simulink model "SysGenBCM_MR0"  (R2015b)
settings: Solver=ode45  StartTime=0.0  StopTime=2e-3  MaxStep=100e-6  RelTol=1e-3
undefined symbols (not defined in the file): AXI4, Lite
libraries: xbsIndex_r4 x89
settings Model: DataTypeOverride=Double  MinMaxOverflowLogging=MinMaxAndOverflow  FPTRunName=DoubleOverride  Creator=ssmith  LastModifiedBy=leosap
settings DataIOCC: SaveFormat=Array
settings DebuggingCC: UnderspecifiedInitializationDetection=Classic  MergeDetectMultiDrivingBlocksExec=none  SolverPrmCheckMsg=warning
settings HardwareCC: ProdBitPerPointer=32  ProdLargestAtomicFloat=None  ProdIntDivRoundTo=Undefined  ProdEndianess=Unspecified  ProdWordSize=32  ProdHWDeviceType=32-bit Generic
settings GRTTargetCC: GeneratePreprocessorConditionals=Disable all
settings ConfigComp: CovModelRefEnable=Off  CovSFcnEnable=off

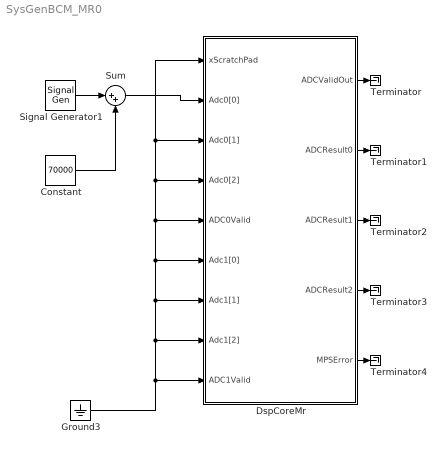
== system SysGenBCM_MR0 ==
  Constant : Constant  Value=70000
  DspCoreMr : Subsystem
  Ground3 : Ground
  Signal Generator1 : SignalGenerator  Amplitude=65000  Frequency=1E+6  Units=rad/sec
  Sum : Sum  Inputs=|++
  Terminator{,1..4} (5 alike) : Terminator
  wires:
  Ground3/1 -> DspCoreMr/9(ADC1Valid), DspCoreMr/8(Adc1[2]), DspCoreMr/7(Adc1[1]), DspCoreMr/6(Adc1[0]), DspCoreMr/3(Adc0[1]), DspCoreMr/1(xScratchPad), DspCoreMr/4(Adc0[2]), DspCoreMr/5(ADC0Valid)
  Constant/1 -> Sum/2
  Signal Generator1/1 -> Sum/1
  Sum/1 -> DspCoreMr/2(Adc0[0])
  DspCoreMr/1(ADCValidOut) -> Terminator/1
  DspCoreMr/2(ADCResult0) -> Terminator1/1
  DspCoreMr/3(ADCResult1) -> Terminator2/1
  DspCoreMr/4(ADCResult2) -> Terminator3/1
  DspCoreMr/5(MPSError) -> Terminator4/1

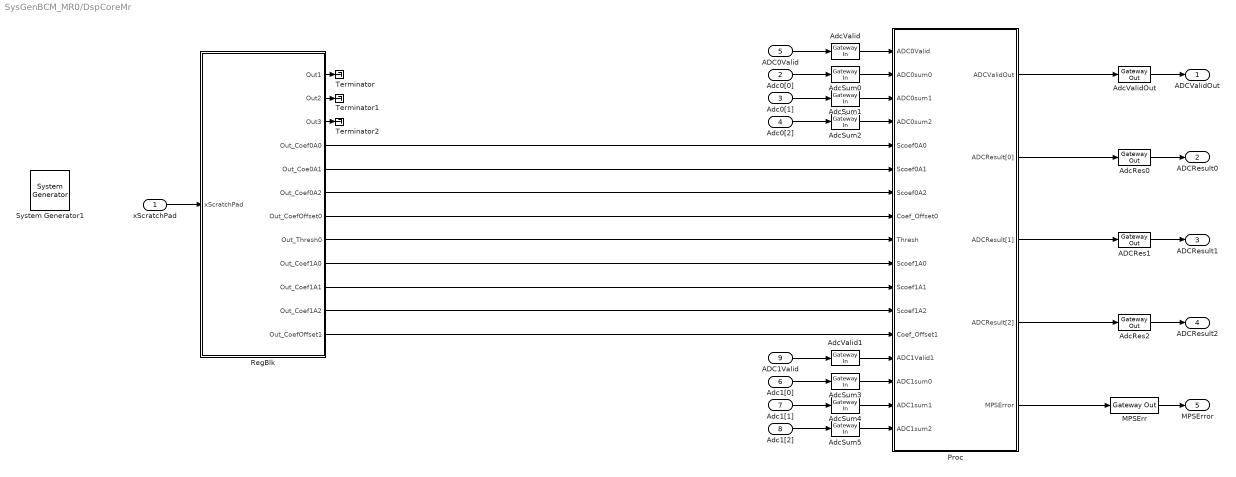
== system SysGenBCM_MR0/DspCoreMr ==
  xScratchPad : Inport
  Adc0[0] : Inport  Port=2
  Adc0[1] : Inport  Port=3
  Adc0[2] : Inport  Port=4
  ADC0Valid : Inport  Port=5
  Adc1[0] : Inport  Port=6
  Adc1[1] : Inport  Port=7
  Adc1[2] : Inport  Port=8
  ADC1Valid : Inport  Port=9
  " System Generator1" : xbsIndex_r4/ System Generator  Tag=genX  xilinxfamily=kintexu  part=xcku040  speed=-2-e  package=ffva1156  synthesis_tool=Vivado  clock_wrapper=Clock Enables  directory=./netlist  proj_type=Vivado  Synth_file=Vivado Synthesis Defaults  Impl_file=Vivado Implementation Defaults  testbench=off  simulink_period=5.385e-9  sysclk_period=5.385  dcm_input_clock_period=10  incr_netlist=off  trim_vbits=Everywhere in SubSystem  dbl_ovrd=According to Block Masks  core_generation=According to Block Masks  run_coregen=off  deprecated_control=off  eval_field=0  block_type=sysgen
  ADCRes1 : xbsIndex_r4/Gateway Out  inherit_from_input=on  hdl_port=on  rows=1  columns=1  UseAsDAC=off  DACChannel='1'  interface=None  automatic_assignment=on  address_offset=hex2dec('00')  intf_name=''  intf_description=''  timing_constraint=None  locs_specified=off  LOCs={}  io_standard={}  block_type=gatewayout
  AdcRes0 : xbsIndex_r4/Gateway Out  inherit_from_input=on  hdl_port=on  rows=1  columns=1  UseAsDAC=off  DACChannel='1'  interface=None  automatic_assignment=on  address_offset=hex2dec('00')  intf_name=''  intf_description=''  timing_constraint=None  locs_specified=off  LOCs={}  io_standard={}  block_type=gatewayout
  AdcRes2 : xbsIndex_r4/Gateway Out  inherit_from_input=on  hdl_port=on  rows=1  columns=1  UseAsDAC=off  DACChannel='1'  interface=None  automatic_assignment=on  address_offset=hex2dec('00')  intf_name=''  intf_description=''  timing_constraint=None  locs_specified=off  LOCs={}  io_standard={}  block_type=gatewayout
  AdcSum{0..5} (6 alike) : xbsIndex_r4/Gateway In  gui_display_data_type=Fixed-point  arith_type=Unsigned  n_bits=32  bin_pt=0  preci_type=Single  exp_width=8  frac_width=24  rows=1  columns=1  quantization="Round  (unbiased: +/- Inf)"  overflow=Saturate  period=5.385E-9  UseAsADC=off  ADCChannel='1'  interface=None  automatic_assignment=on  address_offset=hex2dec('00')  intf_name=''  intf_description=''  default_value=0  timing_constraint=None  locs_specified=off  LOCs={}  io_standard={}  inherit_from_input=off  hdl_port=on  dbl_ovrd=off  block_type=gatewayin
  AdcValid : xbsIndex_r4/Gateway In  gui_display_data_type=Boolean  arith_type=Boolean  n_bits=1  bin_pt=0  preci_type=Single  exp_width=8  frac_width=24  rows=1  columns=1  quantization="Round  (unbiased: +/- Inf)"  overflow=Saturate  period=5.385E-9  UseAsADC=off  ADCChannel='1'  interface=None  automatic_assignment=on  address_offset=hex2dec('00')  intf_name=''  intf_description=''  default_value=0  timing_constraint=None  locs_specified=off  LOCs={}  io_standard={}  inherit_from_input=off  hdl_port=on  dbl_ovrd=off  block_type=gatewayin
  AdcValid1 : xbsIndex_r4/Gateway In  gui_display_data_type=Boolean  arith_type=Boolean  n_bits=1  bin_pt=0  preci_type=Single  exp_width=8  frac_width=24  rows=1  columns=1  quantization="Round  (unbiased: +/- Inf)"  overflow=Saturate  period=5.385E-9  UseAsADC=off  ADCChannel='1'  interface=None  automatic_assignment=on  address_offset=hex2dec('00')  intf_name=''  intf_description=''  default_value=0  timing_constraint=None  locs_specified=off  LOCs={}  io_standard={}  inherit_from_input=off  hdl_port=on  dbl_ovrd=off  block_type=gatewayin
  AdcValidOut : xbsIndex_r4/Gateway Out  inherit_from_input=on  hdl_port=on  rows=1  columns=1  UseAsDAC=off  DACChannel='1'  interface=None  automatic_assignment=on  address_offset=hex2dec('00')  intf_name=''  intf_description=''  timing_constraint=None  locs_specified=off  LOCs={}  io_standard={}  block_type=gatewayout
  MPSErr : xbsIndex_r4/Gateway Out  inherit_from_input=on  hdl_port=on  rows=1  columns=1  UseAsDAC=off  DACChannel='1'  interface=None  automatic_assignment=on  address_offset=hex2dec('00')  intf_name=''  intf_description=''  timing_constraint=None  locs_specified=off  LOCs={}  io_standard={}  block_type=gatewayout
  Proc : Subsystem
  RegBlk : Subsystem
  Terminator : Terminator
  Terminator1 : Terminator
  Terminator2 : Terminator
  ADCValidOut : Outport
  ADCResult0 : Outport  Port=2
  ADCResult1 : Outport  Port=3
  ADCResult2 : Outport  Port=4
  MPSError : Outport  Port=5
  wires:
  xScratchPad/1 -> RegBlk/1(xScratchPad)
  Proc/1(ADCValidOut) -> AdcValidOut/1
  Adc0[2]/1 -> AdcSum2/1
  Adc0[1]/1 -> AdcSum1/1
  Adc0[0]/1 -> AdcSum0/1
  Proc/3(ADCResult[1]) -> ADCRes1/1
  Proc/4(ADCResult[2]) -> AdcRes2/1
  Proc/2(ADCResult[0]) -> AdcRes0/1
  ADC0Valid/1 -> AdcValid/1
  AdcRes0/1 -> ADCResult0/1
  AdcRes2/1 -> ADCResult2/1
  ADCRes1/1 -> ADCResult1/1
  AdcValidOut/1 -> ADCValidOut/1
  AdcValid/1 -> Proc/1(ADC0Valid)
  AdcSum2/1 -> Proc/4(ADC0sum2)
  AdcSum1/1 -> Proc/3(ADC0sum1)
  AdcSum0/1 -> Proc/2(ADC0sum0)
  MPSErr/1 -> MPSError/1
  Adc1[2]/1 -> AdcSum5/1
  Adc1[1]/1 -> AdcSum4/1
  Adc1[0]/1 -> AdcSum3/1
  ADC1Valid/1 -> AdcValid1/1
  AdcValid1/1 -> Proc/14(ADC1Valid1)
  AdcSum5/1 -> Proc/17(ADC1sum2)
  AdcSum4/1 -> Proc/16(ADC1sum1)
  AdcSum3/1 -> Proc/15("ADC1sum0 ")
  RegBlk/4(Out_Coef0A0) -> Proc/5(Scoef0A0)
  RegBlk/12(Out_CoefOffset1) -> Proc/13(Coef_Offset1)
  RegBlk/5(Out_Coe0A1) -> Proc/6(Scoef0A1)
  RegBlk/6(Out_Coef0A2) -> Proc/7(Scoef0A2)
  RegBlk/7(Out_CoefOffset0) -> Proc/8(Coef_Offset0)
  RegBlk/8(Out_Thresh0) -> Proc/9(Thresh)
  RegBlk/9(Out_Coef1A0) -> Proc/10("Scoef1A0 ")
  RegBlk/10(Out_Coef1A1) -> Proc/11(Scoef1A1)
  RegBlk/11(Out_Coef1A2) -> Proc/12(Scoef1A2)
  RegBlk/1(Out1) -> Terminator/1
  RegBlk/2(Out2) -> Terminator1/1
  RegBlk/3(Out3) -> Terminator2/1
  Proc/5(MPSError) -> MPSErr/1

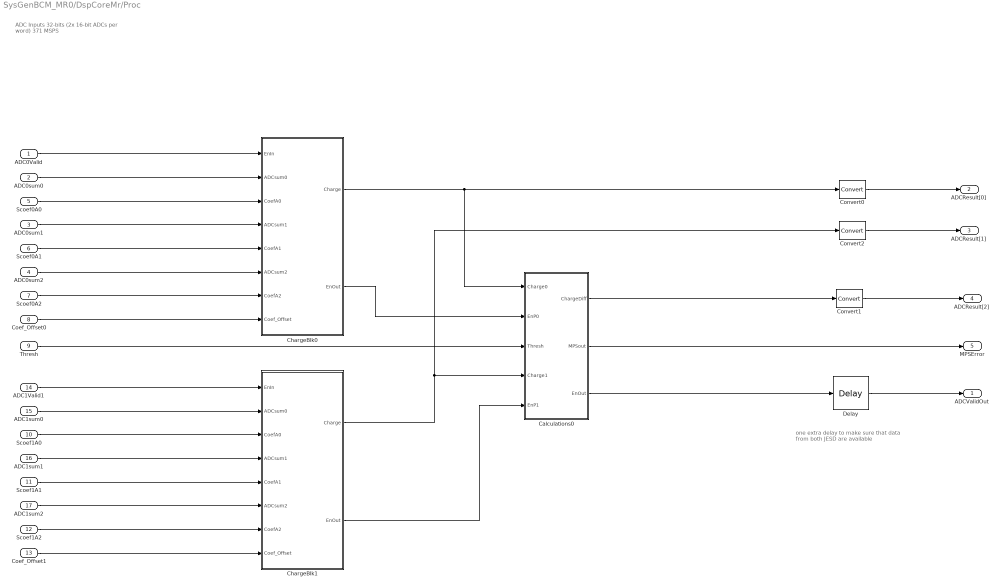
== system SysGenBCM_MR0/DspCoreMr/Proc ==
  note: ADC Inputs
      | 32-bits (2x 16-bit ADCs per word)
      | 371 MSPS
  note: one extra delay to make sure that data from both JESD are available
  ADC0Valid : Inport
  ADC0sum0 : Inport  Port=2
  ADC0sum1 : Inport  Port=3
  ADC0sum2 : Inport  Port=4
  Scoef0A0 : Inport  Port=5  SampleTime=5.385E-9
  Scoef0A1 : Inport  Port=6  SampleTime=5.385E-9
  Scoef0A2 : Inport  Port=7  SampleTime=5.385E-9
  Coef_Offset0 : Inport  Port=8  SampleTime=5.385E-9
  Thresh : Inport  Port=9  SampleTime=5.385E-9
  "Scoef1A0 " : Inport  Port=10  SampleTime=5.385E-9
  Scoef1A1 : Inport  Port=11  SampleTime=5.385E-9
  Scoef1A2 : Inport  Port=12  SampleTime=5.385E-9
  Coef_Offset1 : Inport  Port=13  SampleTime=5.385E-9
  ADC1Valid1 : Inport  Port=14
  "ADC1sum0 " : Inport  Port=15
  ADC1sum1 : Inport  Port=16
  ADC1sum2 : Inport  Port=17
  Calculations0 : Subsystem
  ChargeBlk0 : Subsystem
  ChargeBlk1 : Subsystem
  Convert0 : xbsIndex_r4/Convert  gui_display_data_type=Fixed-point  arith_type="Signed  (2's comp)"  n_bits=32  bin_pt=0  float_type=Single  exp_bits=8  fraction_bits=24  quantization="Round  (unbiased: +/- Inf)"  overflow=Saturate  en=off  latency=1  pipeline=off  dbl_ovrd=off  block_type=convert
  Convert1 : xbsIndex_r4/Convert  gui_display_data_type=Fixed-point  arith_type="Signed  (2's comp)"  n_bits=32  bin_pt=0  float_type=Single  exp_bits=8  fraction_bits=24  quantization="Round  (unbiased: +/- Inf)"  overflow=Saturate  en=off  latency=1  pipeline=off  dbl_ovrd=off  block_type=convert
  Convert2 : xbsIndex_r4/Convert  gui_display_data_type=Fixed-point  arith_type="Signed  (2's comp)"  n_bits=32  bin_pt=0  float_type=Single  exp_bits=8  fraction_bits=24  quantization="Round  (unbiased: +/- Inf)"  overflow=Saturate  en=off  latency=1  pipeline=off  dbl_ovrd=off  block_type=convert
  Delay : xbsIndex_r4/Delay  rst=off  infoeditControl=Selection of Reset will increase slice count due to use of real FFs and instead of SRLs  en=off  latency=2  reg_retiming=off  dbl_ovrd=off  block_type=delay
      settings: infoedit=Hardware notes: A delay line is a chain, each link of which is an SRL16 or SRL32 followed by a flip-flop.
  ADCValidOut : Outport
  ADCResult[0] : Outport  Port=2
  ADCResult[1] : Outport  Port=3
  ADCResult[2] : Outport  Port=4
  MPSError : Outport  Port=5
  wires:
  Convert0/1 -> ADCResult[0]/1
  Convert1/1 -> ADCResult[2]/1
  Delay/1 -> ADCValidOut/1
  Convert2/1 -> ADCResult[1]/1
  Calculations0/1(ChargeDiff) -> Convert1/1
  Calculations0/3(EnOut) -> Delay/1
  Calculations0/2(MPSout) -> MPSError/1
  Thresh/1 -> Calculations0/3(Thresh)
  ADC0Valid/1 -> ChargeBlk0/1(EnIn)
  ADC0sum0/1 -> ChargeBlk0/2(ADCsum0)
  Scoef0A0/1 -> ChargeBlk0/3(CoefA0)
  ADC0sum1/1 -> ChargeBlk0/4(ADCsum1)
  Scoef0A1/1 -> ChargeBlk0/5(CoefA1)
  ADC0sum2/1 -> ChargeBlk0/6(ADCsum2)
  Scoef0A2/1 -> ChargeBlk0/7(CoefA2)
  Coef_Offset0/1 -> ChargeBlk0/8(Coef_Offset)
  ChargeBlk0/2(EnOut) -> Calculations0/2(EnP0)
  ChargeBlk0/1(Charge) -> Calculations0/1(Charge0), Convert0/1
  ChargeBlk1/1(Charge) -> Convert2/1, Calculations0/4(Charge1)
  ChargeBlk1/2(EnOut) -> Calculations0/5(EnP1)
  ADC1Valid1/1 -> ChargeBlk1/1(EnIn)
  "ADC1sum0 "/1 -> ChargeBlk1/2(ADCsum0)
  "Scoef1A0 "/1 -> ChargeBlk1/3(CoefA0)
  ADC1sum1/1 -> ChargeBlk1/4(ADCsum1)
  Scoef1A1/1 -> ChargeBlk1/5(CoefA1)
  ADC1sum2/1 -> ChargeBlk1/6(ADCsum2)
  Scoef1A2/1 -> ChargeBlk1/7(CoefA2)
  Coef_Offset1/1 -> ChargeBlk1/8(Coef_Offset)

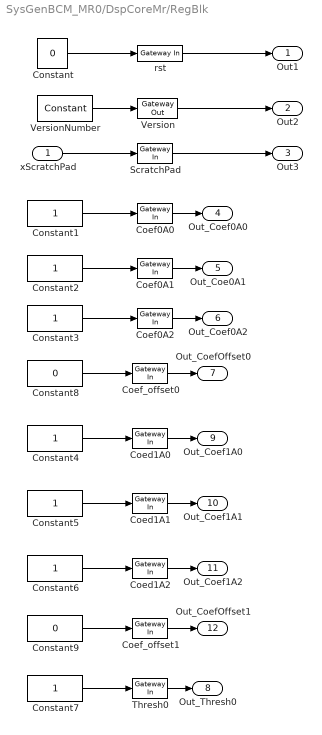
== system SysGenBCM_MR0/DspCoreMr/RegBlk ==
  xScratchPad : Inport
  Coed1A0 : xbsIndex_r4/Gateway In  gui_display_data_type=Floating-point  arith_type=Floating-point  n_bits=32  bin_pt=0  preci_type=Single  exp_width=8  frac_width=24  rows=1  columns=1  quantization="Round  (unbiased: +/- Inf)"  overflow=Saturate  period=5.385E-9  UseAsADC=off  ADCChannel='1'  interface=AXI4-Lite  automatic_assignment=off  address_offset=hex2dec('014')  intf_name='rwreg'  intf_description=''  default_value=0  timing_constraint=None  locs_specified=off  LOCs={}  io_standard={}  inherit_from_input=off  hdl_port=on  dbl_ovrd=off  block_type=gatewayin
  Coed1A1 : xbsIndex_r4/Gateway In  gui_display_data_type=Floating-point  arith_type=Floating-point  n_bits=32  bin_pt=0  preci_type=Single  exp_width=8  frac_width=24  rows=1  columns=1  quantization="Round  (unbiased: +/- Inf)"  overflow=Saturate  period=5.385E-9  UseAsADC=off  ADCChannel='1'  interface=AXI4-Lite  automatic_assignment=off  address_offset=hex2dec('018')  intf_name='rwreg'  intf_description=''  default_value=0  timing_constraint=None  locs_specified=off  LOCs={}  io_standard={}  inherit_from_input=off  hdl_port=on  dbl_ovrd=off  block_type=gatewayin
  Coed1A2 : xbsIndex_r4/Gateway In  gui_display_data_type=Floating-point  arith_type=Floating-point  n_bits=32  bin_pt=0  preci_type=Single  exp_width=8  frac_width=24  rows=1  columns=1  quantization="Round  (unbiased: +/- Inf)"  overflow=Saturate  period=5.385E-9  UseAsADC=off  ADCChannel='1'  interface=AXI4-Lite  automatic_assignment=off  address_offset=hex2dec('01C')  intf_name='rwreg'  intf_description=''  default_value=0  timing_constraint=None  locs_specified=off  LOCs={}  io_standard={}  inherit_from_input=off  hdl_port=on  dbl_ovrd=off  block_type=gatewayin
  Coef0A0 : xbsIndex_r4/Gateway In  gui_display_data_type=Floating-point  arith_type=Floating-point  n_bits=32  bin_pt=31  preci_type=Single  exp_width=8  frac_width=24  rows=1  columns=1  quantization="Round  (unbiased: +/- Inf)"  overflow=Saturate  period=5.385E-9  UseAsADC=off  ADCChannel='1'  interface=AXI4-Lite  automatic_assignment=off  address_offset=hex2dec('004')  intf_name='rwreg'  intf_description=''  default_value=hex2dec('3f800000')  timing_constraint=None  locs_specified=off  LOCs={}  io_standard={}  inherit_from_input=off  hdl_port=on  dbl_ovrd=off  block_type=gatewayin
  Coef0A1 : xbsIndex_r4/Gateway In  gui_display_data_type=Floating-point  arith_type=Floating-point  n_bits=32  bin_pt=0  preci_type=Single  exp_width=8  frac_width=24  rows=1  columns=1  quantization="Round  (unbiased: +/- Inf)"  overflow=Saturate  period=5.385E-9  UseAsADC=off  ADCChannel='1'  interface=AXI4-Lite  automatic_assignment=off  address_offset=hex2dec('008')  intf_name='rwreg'  intf_description=''  default_value=hex2dec('3f800001')  timing_constraint=None  locs_specified=off  LOCs={}  io_standard={}  inherit_from_input=off  hdl_port=on  dbl_ovrd=off  block_type=gatewayin
  Coef0A2 : xbsIndex_r4/Gateway In  gui_display_data_type=Floating-point  arith_type=Floating-point  n_bits=32  bin_pt=0  preci_type=Single  exp_width=8  frac_width=24  rows=1  columns=1  quantization="Round  (unbiased: +/- Inf)"  overflow=Saturate  period=5.385E-9  UseAsADC=off  ADCChannel='1'  interface=AXI4-Lite  automatic_assignment=off  address_offset=hex2dec('00C')  intf_name='rwreg'  intf_description=''  default_value=hex2dec('3f800002')  timing_constraint=None  locs_specified=off  LOCs={}  io_standard={}  inherit_from_input=off  hdl_port=on  dbl_ovrd=off  block_type=gatewayin
  Coef_offset0 : xbsIndex_r4/Gateway In  gui_display_data_type=Floating-point  arith_type=Floating-point  n_bits=32  bin_pt=0  preci_type=Single  exp_width=8  frac_width=24  rows=1  columns=1  quantization="Round  (unbiased: +/- Inf)"  overflow=Saturate  period=5.385E-9  UseAsADC=off  ADCChannel='1'  interface=AXI4-Lite  automatic_assignment=off  address_offset=hex2dec('010')  intf_name='rwreg'  intf_description=''  default_value=0  timing_constraint=None  locs_specified=off  LOCs={}  io_standard={}  inherit_from_input=off  hdl_port=on  dbl_ovrd=off  block_type=gatewayin
  Coef_offset1 : xbsIndex_r4/Gateway In  gui_display_data_type=Floating-point  arith_type=Floating-point  n_bits=32  bin_pt=0  preci_type=Single  exp_width=8  frac_width=24  rows=1  columns=1  quantization="Round  (unbiased: +/- Inf)"  overflow=Saturate  period=5.385E-9  UseAsADC=off  ADCChannel='1'  interface=AXI4-Lite  automatic_assignment=off  address_offset=hex2dec('020')  intf_name='rwreg'  intf_description=''  default_value=0  timing_constraint=None  locs_specified=off  LOCs={}  io_standard={}  inherit_from_input=off  hdl_port=on  dbl_ovrd=off  block_type=gatewayin
  Constant : Constant  Value=0
  Constant{1..7} (7 alike) : Constant
  Constant8 : Constant  Value=0
  Constant9 : Constant  Value=0
  ScratchPad : xbsIndex_r4/Gateway In  gui_display_data_type=Fixed-point  arith_type="Signed  (2's comp)"  n_bits=32  bin_pt=0  preci_type=Single  exp_width=8  frac_width=24  rows=1  columns=1  quantization="Round  (unbiased: +/- Inf)"  overflow=Saturate  period=5.385e-9  UseAsADC=off  ADCChannel='1'  interface=AXI4-Lite  automatic_assignment=off  address_offset=hex2dec('FFC')  intf_name=''  intf_description=''  default_value=0  timing_constraint=None  locs_specified=off  LOCs={}  io_standard={}  inherit_from_input=off  hdl_port=on  dbl_ovrd=off  block_type=gatewayin
  Thresh0 : xbsIndex_r4/Gateway In  gui_display_data_type=Floating-point  arith_type=Floating-point  n_bits=32  bin_pt=0  preci_type=Single  exp_width=8  frac_width=24  rows=1  columns=1  quantization="Round  (unbiased: +/- Inf)"  overflow=Saturate  period=5.385E-9  UseAsADC=off  ADCChannel='1'  interface=AXI4-Lite  automatic_assignment=off  address_offset=hex2dec('024')  intf_name='rwreg'  intf_description=''  default_value=0  timing_constraint=None  locs_specified=off  LOCs={}  io_standard={}  inherit_from_input=off  hdl_port=on  dbl_ovrd=off  block_type=gatewayin
  Version : xbsIndex_r4/Gateway Out  inherit_from_input=on  hdl_port=on  rows=1  columns=1  UseAsDAC=off  DACChannel='1'  interface=AXI4-Lite  automatic_assignment=off  address_offset=hex2dec('000')  intf_name='rwreg'  intf_description=''  timing_constraint=None  locs_specified=off  LOCs={}  io_standard={}  block_type=gatewayout
  VersionNumber : xbsIndex_r4/Constant  const=hex2dec('00000001')  gui_display_data_type=Fixed-point  arith_type=Unsigned  n_bits=32  bin_pt=0  preci_type=Single  exp_width=8  frac_width=24  explicit_period=off  period=1  equ=P=C  opselect=C  inp2=PCIN>>17  opr=+  inp1=P  carry=CIN  dbl_ovrd=off  block_type=constant
  rst : xbsIndex_r4/Gateway In  gui_display_data_type=Boolean  arith_type=Boolean  n_bits=16  bin_pt=14  preci_type=Single  exp_width=8  frac_width=24  rows=1  columns=1  quantization="Round  (unbiased: +/- Inf)"  overflow=Saturate  period=5.385e-9  UseAsADC=off  ADCChannel='1'  interface=None  automatic_assignment=on  address_offset=hex2dec('00')  intf_name=''  intf_description=''  default_value=0  timing_constraint=None  locs_specified=off  LOCs={}  io_standard={}  inherit_from_input=off  hdl_port=on  dbl_ovrd=off  block_type=gatewayin
  Out1 : Outport
  Out2 : Outport  Port=2
  Out3 : Outport  Port=3
  Out_Coef0A0 : Outport  Port=4
  Out_Coe0A1 : Outport  Port=5
  Out_Coef0A2 : Outport  Port=6
  Out_CoefOffset0 : Outport  Port=7
  Out_Thresh0 : Outport  Port=8
  Out_Coef1A0 : Outport  Port=9
  Out_Coef1A1 : Outport  Port=10
  Out_Coef1A2 : Outport  Port=11
  Out_CoefOffset1 : Outport  Port=12
  wires:
  Constant/1 -> rst/1
  ScratchPad/1 -> Out3/1
  Version/1 -> Out2/1
  rst/1 -> Out1/1
  xScratchPad/1 -> ScratchPad/1
  VersionNumber/1 -> Version/1
  Constant1/1 -> Coef0A0/1
  Coef0A0/1 -> Out_Coef0A0/1
  Constant2/1 -> Coef0A1/1
  Coef0A1/1 -> Out_Coe0A1/1
  Constant3/1 -> Coef0A2/1
  Coef0A2/1 -> Out_Coef0A2/1
  Constant4/1 -> Coed1A0/1
  Coed1A0/1 -> Out_Coef1A0/1
  Constant5/1 -> Coed1A1/1
  Constant6/1 -> Coed1A2/1
  Constant7/1 -> Thresh0/1
  Coed1A2/1 -> Out_Coef1A2/1
  Coed1A1/1 -> Out_Coef1A1/1
  Thresh0/1 -> Out_Thresh0/1
  Constant8/1 -> Coef_offset0/1
  Coef_offset0/1 -> Out_CoefOffset0/1
  Constant9/1 -> Coef_offset1/1
  Coef_offset1/1 -> Out_CoefOffset1/1

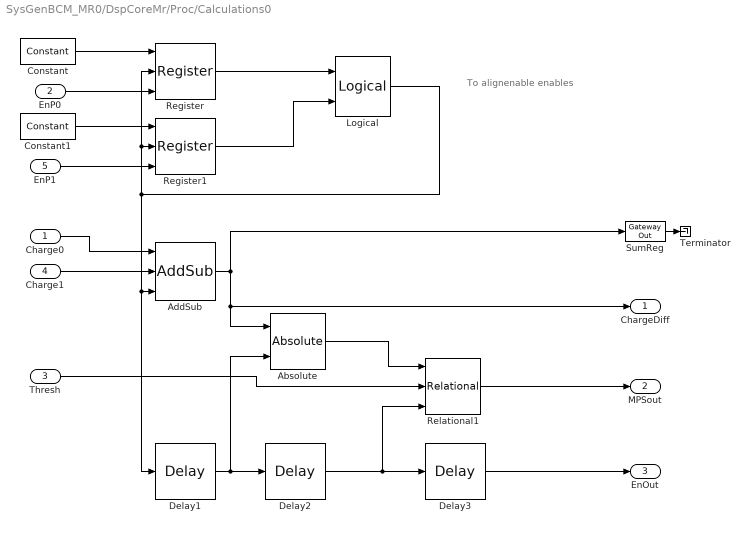
== system SysGenBCM_MR0/DspCoreMr/Proc/Calculations0 ==
  note: To alignenable enables
  Charge0 : Inport
  EnP0 : Inport  Port=2
  Thresh : Inport  Port=3
  Charge1 : Inport  Port=4
  EnP1 : Inport  Port=5
  Absolute : xbsIndex_r4/Absolute  precision=Full  arith_type=Unsigned  n_bits=16  bin_pt=14  quantization=Truncate  overflow=Wrap  en=on  latency=1  dbl_ovrd=off  block_type=abs
  AddSub : xbsIndex_r4/AddSub  mode=Subtraction  use_carryin=off  use_carryout=off  en=on  latency=3  precision=Full  arith_type=Unsigned  n_bits=16  bin_pt=14  quantization=Truncate  overflow=Wrap  use_behavioral_HDL=off  hw_selection=Fabric  pipelined=off  dbl_ovrd=off  block_type=addsub
  Constant : xbsIndex_r4/Constant  const=1.0  gui_display_data_type=Boolean  arith_type=Boolean  n_bits=16  bin_pt=14  preci_type=Single  exp_width=8  frac_width=24  explicit_period=off  period=1  equ=P=C  opselect=C  inp2=PCIN>>17  opr=+  inp1=P  carry=CIN  dbl_ovrd=off  block_type=constant
  Constant1 : xbsIndex_r4/Constant  const=1.0  gui_display_data_type=Boolean  arith_type=Boolean  n_bits=16  bin_pt=14  preci_type=Single  exp_width=8  frac_width=24  explicit_period=off  period=1  equ=P=C  opselect=C  inp2=PCIN>>17  opr=+  inp1=P  carry=CIN  dbl_ovrd=off  block_type=constant
  Delay1 : xbsIndex_r4/Delay  rst=off  infoeditControl=Selection of Reset will increase slice count due to use of real FFs and instead of SRLs  en=off  latency=3  reg_retiming=off  dbl_ovrd=off  block_type=delay
      settings: infoedit=Hardware notes: A delay line is a chain, each link of which is an SRL16 or SRL32 followed by a flip-flop.
  Delay2 : xbsIndex_r4/Delay  rst=off  infoeditControl=Selection of Reset will increase slice count due to use of real FFs and instead of SRLs  en=off  latency=1  reg_retiming=off  dbl_ovrd=off  block_type=delay
      settings: infoedit=Hardware notes: A delay line is a chain, each link of which is an SRL16 or SRL32 followed by a flip-flop.
  Delay3 : xbsIndex_r4/Delay  rst=off  infoeditControl=Selection of Reset will increase slice count due to use of real FFs and instead of SRLs  en=off  latency=1  reg_retiming=off  dbl_ovrd=off  block_type=delay
      settings: infoedit=Hardware notes: A delay line is a chain, each link of which is an SRL16 or SRL32 followed by a flip-flop.
  Logical : xbsIndex_r4/Logical  logical_function=AND  inputs=2  en=off  latency=0  precision=Full  arith_type=Unsigned  n_bits=16  bin_pt=0  align_bp=on  dbl_ovrd=off  block_type=logical
  Register : xbsIndex_r4/Register  init=0  rst=on  en=on  dbl_ovrd=off  block_type=register
  Register1 : xbsIndex_r4/Register  init=0  rst=on  en=on  dbl_ovrd=off  block_type=register
  Relational1 : xbsIndex_r4/Relational  mode=a>=b  op_type=Bool  en=on  latency=1  dbl_ovrd=off  block_type=relational
  SumReg : xbsIndex_r4/Gateway Out  inherit_from_input=on  hdl_port=on  rows=1  columns=1  UseAsDAC=off  DACChannel='1'  interface=AXI4-Lite  automatic_assignment=off  address_offset=hex2dec('130')  intf_name=''  intf_description=''  timing_constraint=None  locs_specified=off  LOCs={}  io_standard={}  block_type=gatewayout
  Terminator : Terminator
  ChargeDiff : Outport
  MPSout : Outport  Port=2
  EnOut : Outport  Port=3
  wires:
  AddSub/1 -> SumReg/1, ChargeDiff/1, Absolute/1
  Delay1/1 -> Absolute/2, Delay2/1
  Charge1/1 -> AddSub/2
  Charge0/1 -> AddSub/1
  SumReg/1 -> Terminator/1
  Absolute/1 -> Relational1/1
  Delay2/1 -> Relational1/3, Delay3/1
  Thresh/1 -> Relational1/2
  Delay3/1 -> EnOut/1
  Relational1/1 -> MPSout/1
  Constant/1 -> Register/1
  Register/1 -> Logical/1
  Constant1/1 -> Register1/1
  Register1/1 -> Logical/2
  Logical/1 -> Register/2, Register1/2, Delay1/1, AddSub/3
  EnP1/1 -> Register1/3
  EnP0/1 -> Register/3

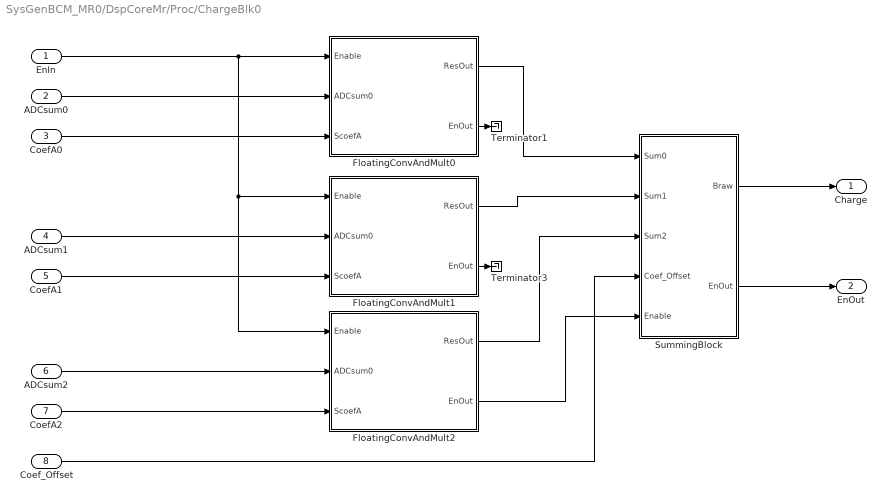
== system SysGenBCM_MR0/DspCoreMr/Proc/ChargeBlk0 ==
  EnIn : Inport
  ADCsum0 : Inport  Port=2
  CoefA0 : Inport  Port=3
  ADCsum1 : Inport  Port=4
  CoefA1 : Inport  Port=5
  ADCsum2 : Inport  Port=6
  CoefA2 : Inport  Port=7
  Coef_Offset : Inport  Port=8
  FloatingConvAndMult0 : Subsystem
  FloatingConvAndMult1 : Subsystem
  FloatingConvAndMult2 : Subsystem
  SummingBlock : Subsystem
  Terminator1 : Terminator
  Terminator3 : Terminator
  Charge : Outport
  EnOut : Outport  Port=2
  wires:
  SummingBlock/2(EnOut) -> EnOut/1
  FloatingConvAndMult2/2(EnOut) -> SummingBlock/5(Enable)
  Coef_Offset/1 -> SummingBlock/4(Coef_Offset)
  FloatingConvAndMult1/2(EnOut) -> Terminator3/1
  FloatingConvAndMult0/2(EnOut) -> Terminator1/1
  FloatingConvAndMult2/1(ResOut) -> SummingBlock/3(Sum2)
  EnIn/1 -> FloatingConvAndMult2/1(Enable), FloatingConvAndMult1/1(Enable), FloatingConvAndMult0/1(Enable)
  ADCsum2/1 -> FloatingConvAndMult2/2(ADCsum0)
  ADCsum1/1 -> FloatingConvAndMult1/2(ADCsum0)
  ADCsum0/1 -> FloatingConvAndMult0/2(ADCsum0)
  FloatingConvAndMult1/1(ResOut) -> SummingBlock/2(Sum1)
  FloatingConvAndMult0/1(ResOut) -> SummingBlock/1(Sum0)
  CoefA2/1 -> FloatingConvAndMult2/3(ScoefA)
  CoefA1/1 -> FloatingConvAndMult1/3(ScoefA)
  CoefA0/1 -> FloatingConvAndMult0/3(ScoefA)
  SummingBlock/1(Braw) -> Charge/1

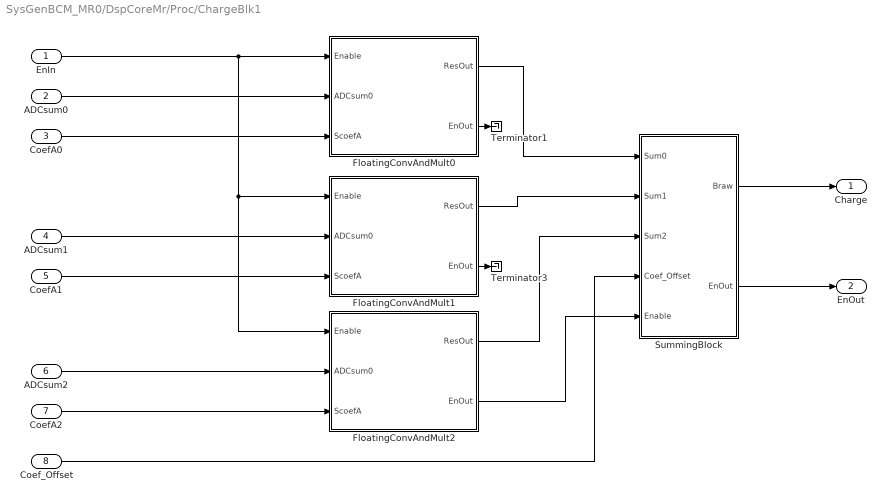
== system SysGenBCM_MR0/DspCoreMr/Proc/ChargeBlk1 ==
  EnIn : Inport
  ADCsum0 : Inport  Port=2
  CoefA0 : Inport  Port=3
  ADCsum1 : Inport  Port=4
  CoefA1 : Inport  Port=5
  ADCsum2 : Inport  Port=6
  CoefA2 : Inport  Port=7
  Coef_Offset : Inport  Port=8
  FloatingConvAndMult0 : Subsystem
  FloatingConvAndMult1 : Subsystem
  FloatingConvAndMult2 : Subsystem
  SummingBlock : Subsystem
  Terminator1 : Terminator
  Terminator3 : Terminator
  Charge : Outport
  EnOut : Outport  Port=2
  wires:
  SummingBlock/2(EnOut) -> EnOut/1
  FloatingConvAndMult2/2(EnOut) -> SummingBlock/5(Enable)
  Coef_Offset/1 -> SummingBlock/4(Coef_Offset)
  FloatingConvAndMult1/2(EnOut) -> Terminator3/1
  FloatingConvAndMult0/2(EnOut) -> Terminator1/1
  FloatingConvAndMult2/1(ResOut) -> SummingBlock/3(Sum2)
  EnIn/1 -> FloatingConvAndMult2/1(Enable), FloatingConvAndMult1/1(Enable), FloatingConvAndMult0/1(Enable)
  ADCsum2/1 -> FloatingConvAndMult2/2(ADCsum0)
  ADCsum1/1 -> FloatingConvAndMult1/2(ADCsum0)
  ADCsum0/1 -> FloatingConvAndMult0/2(ADCsum0)
  FloatingConvAndMult1/1(ResOut) -> SummingBlock/2(Sum1)
  FloatingConvAndMult0/1(ResOut) -> SummingBlock/1(Sum0)
  CoefA2/1 -> FloatingConvAndMult2/3(ScoefA)
  CoefA1/1 -> FloatingConvAndMult1/3(ScoefA)
  CoefA0/1 -> FloatingConvAndMult0/3(ScoefA)
  SummingBlock/1(Braw) -> Charge/1

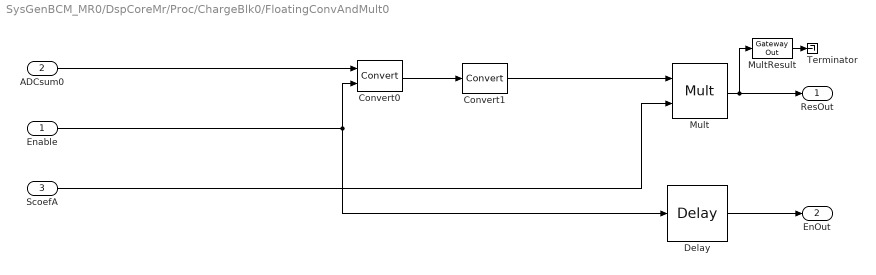
== system SysGenBCM_MR0/DspCoreMr/Proc/ChargeBlk0/FloatingConvAndMult0 ==
  Enable : Inport  SampleTime=5.385E-9
  ADCsum0 : Inport  Port=2
  ScoefA : Inport  Port=3  SampleTime=5.385E-9
  Convert0 : xbsIndex_r4/Convert  gui_display_data_type=Fixed-point  arith_type="Signed  (2's comp)"  n_bits=32  bin_pt=0  float_type=Single  exp_bits=8  fraction_bits=24  quantization=Truncate  overflow=Wrap  en=on  latency=1  pipeline=off  dbl_ovrd=off  block_type=convert
  Convert1 : xbsIndex_r4/Convert  gui_display_data_type=Floating-point  arith_type=Floating-point  n_bits=16  bin_pt=14  float_type=Single  exp_bits=8  fraction_bits=24  quantization=Truncate  overflow=Wrap  en=off  latency=1  pipeline=off  dbl_ovrd=off  block_type=convert
  Delay : xbsIndex_r4/Delay  rst=off  infoeditControl=Selection of Reset will increase slice count due to use of real FFs and instead of SRLs  en=off  latency=6  reg_retiming=off  dbl_ovrd=off  block_type=delay
      settings: infoedit=Hardware notes: A delay line is a chain, each link of which is an SRL16 or SRL32 followed by a flip-flop.
  Mult : xbsIndex_r4/Mult  precision=Full  arith_type="Signed  (2's comp)"  n_bits=16  bin_pt=14  quantization=Truncate  overflow=Wrap  en=off  latency=4  use_behavioral_HDL=off  opt=Speed  use_embedded=on  optimum_pipeline=off  pipeline=on  dbl_ovrd=off  use_rpm=on  placement_style=Triangular  block_type=mult
  MultResult : xbsIndex_r4/Gateway Out  inherit_from_input=on  hdl_port=on  rows=1  columns=1  UseAsDAC=off  DACChannel='1'  interface=AXI4-Lite  automatic_assignment=off  address_offset=hex2dec('100')  intf_name=''  intf_description=''  timing_constraint=None  locs_specified=off  LOCs={}  io_standard={}  block_type=gatewayout
  Terminator : Terminator
  ResOut : Outport
  EnOut : Outport  Port=2
  wires:
  Mult/1 -> MultResult/1, ResOut/1
  Convert0/1 -> Convert1/1
  Enable/1 -> Delay/1, Convert0/2
  ScoefA/1 -> Mult/2
  Convert1/1 -> Mult/1
  Delay/1 -> EnOut/1
  ADCsum0/1 -> Convert0/1
  MultResult/1 -> Terminator/1

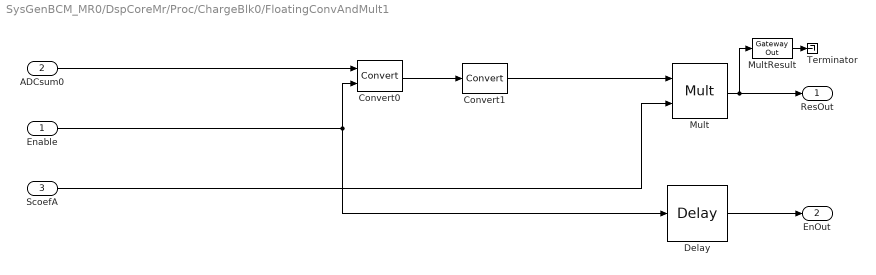
== system SysGenBCM_MR0/DspCoreMr/Proc/ChargeBlk0/FloatingConvAndMult1 ==
  Enable : Inport  SampleTime=5.385E-9
  ADCsum0 : Inport  Port=2
  ScoefA : Inport  Port=3  SampleTime=5.385E-9
  Convert0 : xbsIndex_r4/Convert  gui_display_data_type=Fixed-point  arith_type="Signed  (2's comp)"  n_bits=32  bin_pt=0  float_type=Single  exp_bits=8  fraction_bits=24  quantization=Truncate  overflow=Wrap  en=on  latency=1  pipeline=off  dbl_ovrd=off  block_type=convert
  Convert1 : xbsIndex_r4/Convert  gui_display_data_type=Floating-point  arith_type=Floating-point  n_bits=16  bin_pt=14  float_type=Single  exp_bits=8  fraction_bits=24  quantization=Truncate  overflow=Wrap  en=off  latency=1  pipeline=off  dbl_ovrd=off  block_type=convert
  Delay : xbsIndex_r4/Delay  rst=off  infoeditControl=Selection of Reset will increase slice count due to use of real FFs and instead of SRLs  en=off  latency=6  reg_retiming=off  dbl_ovrd=off  block_type=delay
      settings: infoedit=Hardware notes: A delay line is a chain, each link of which is an SRL16 or SRL32 followed by a flip-flop.
  Mult : xbsIndex_r4/Mult  precision=Full  arith_type="Signed  (2's comp)"  n_bits=16  bin_pt=14  quantization=Truncate  overflow=Wrap  en=off  latency=4  use_behavioral_HDL=off  opt=Speed  use_embedded=on  optimum_pipeline=off  pipeline=on  dbl_ovrd=off  use_rpm=on  placement_style=Triangular  block_type=mult
  MultResult : xbsIndex_r4/Gateway Out  inherit_from_input=on  hdl_port=on  rows=1  columns=1  UseAsDAC=off  DACChannel='1'  interface=AXI4-Lite  automatic_assignment=off  address_offset=hex2dec('104')  intf_name=''  intf_description=''  timing_constraint=None  locs_specified=off  LOCs={}  io_standard={}  block_type=gatewayout
  Terminator : Terminator
  ResOut : Outport
  EnOut : Outport  Port=2
  wires:
  Mult/1 -> MultResult/1, ResOut/1
  Convert0/1 -> Convert1/1
  Enable/1 -> Delay/1, Convert0/2
  ScoefA/1 -> Mult/2
  Convert1/1 -> Mult/1
  Delay/1 -> EnOut/1
  ADCsum0/1 -> Convert0/1
  MultResult/1 -> Terminator/1

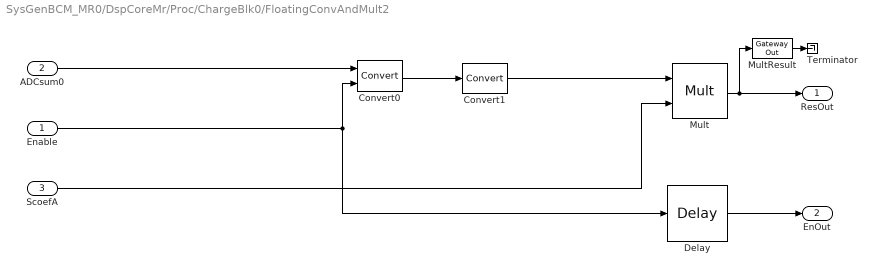
== system SysGenBCM_MR0/DspCoreMr/Proc/ChargeBlk0/FloatingConvAndMult2 ==
  Enable : Inport  SampleTime=5.385E-9
  ADCsum0 : Inport  Port=2
  ScoefA : Inport  Port=3  SampleTime=5.385E-9
  Convert0 : xbsIndex_r4/Convert  gui_display_data_type=Fixed-point  arith_type="Signed  (2's comp)"  n_bits=32  bin_pt=0  float_type=Single  exp_bits=8  fraction_bits=24  quantization=Truncate  overflow=Wrap  en=on  latency=1  pipeline=off  dbl_ovrd=off  block_type=convert
  Convert1 : xbsIndex_r4/Convert  gui_display_data_type=Floating-point  arith_type=Floating-point  n_bits=16  bin_pt=14  float_type=Single  exp_bits=8  fraction_bits=24  quantization=Truncate  overflow=Wrap  en=off  latency=1  pipeline=off  dbl_ovrd=off  block_type=convert
  Delay : xbsIndex_r4/Delay  rst=off  infoeditControl=Selection of Reset will increase slice count due to use of real FFs and instead of SRLs  en=off  latency=6  reg_retiming=off  dbl_ovrd=off  block_type=delay
      settings: infoedit=Hardware notes: A delay line is a chain, each link of which is an SRL16 or SRL32 followed by a flip-flop.
  Mult : xbsIndex_r4/Mult  precision=Full  arith_type="Signed  (2's comp)"  n_bits=16  bin_pt=14  quantization=Truncate  overflow=Wrap  en=off  latency=4  use_behavioral_HDL=off  opt=Speed  use_embedded=on  optimum_pipeline=off  pipeline=on  dbl_ovrd=off  use_rpm=on  placement_style=Triangular  block_type=mult
  MultResult : xbsIndex_r4/Gateway Out  inherit_from_input=on  hdl_port=on  rows=1  columns=1  UseAsDAC=off  DACChannel='1'  interface=AXI4-Lite  automatic_assignment=off  address_offset=hex2dec('108')  intf_name=''  intf_description=''  timing_constraint=None  locs_specified=off  LOCs={}  io_standard={}  block_type=gatewayout
  Terminator : Terminator
  ResOut : Outport
  EnOut : Outport  Port=2
  wires:
  Mult/1 -> MultResult/1, ResOut/1
  Convert0/1 -> Convert1/1
  Enable/1 -> Delay/1, Convert0/2
  ScoefA/1 -> Mult/2
  Convert1/1 -> Mult/1
  Delay/1 -> EnOut/1
  ADCsum0/1 -> Convert0/1
  MultResult/1 -> Terminator/1

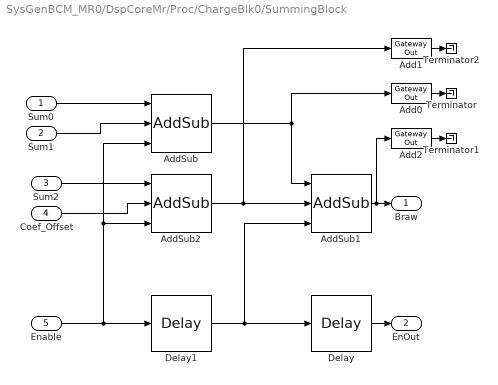
== system SysGenBCM_MR0/DspCoreMr/Proc/ChargeBlk0/SummingBlock ==
  Sum0 : Inport
  Sum1 : Inport  Port=2
  Sum2 : Inport  Port=3
  Coef_Offset : Inport  Port=4
  Enable : Inport  Port=5
  Add0 : xbsIndex_r4/Gateway Out  inherit_from_input=on  hdl_port=on  rows=1  columns=1  UseAsDAC=off  DACChannel='1'  interface=AXI4-Lite  automatic_assignment=off  address_offset=hex2dec('10C')  intf_name=''  intf_description=''  timing_constraint=None  locs_specified=off  LOCs={}  io_standard={}  block_type=gatewayout
  Add1 : xbsIndex_r4/Gateway Out  inherit_from_input=on  hdl_port=on  rows=1  columns=1  UseAsDAC=off  DACChannel='1'  interface=AXI4-Lite  automatic_assignment=off  address_offset=hex2dec('110')  intf_name=''  intf_description=''  timing_constraint=None  locs_specified=off  LOCs={}  io_standard={}  block_type=gatewayout
  Add2 : xbsIndex_r4/Gateway Out  inherit_from_input=on  hdl_port=on  rows=1  columns=1  UseAsDAC=off  DACChannel='1'  interface=AXI4-Lite  automatic_assignment=off  address_offset=hex2dec('114')  intf_name=''  intf_description=''  timing_constraint=None  locs_specified=off  LOCs={}  io_standard={}  block_type=gatewayout
  AddSub : xbsIndex_r4/AddSub  mode=Addition  use_carryin=off  use_carryout=off  en=on  latency=3  precision=Full  arith_type=Unsigned  n_bits=16  bin_pt=14  quantization=Truncate  overflow=Wrap  use_behavioral_HDL=off  hw_selection=Fabric  pipelined=off  dbl_ovrd=off  block_type=addsub
  AddSub1 : xbsIndex_r4/AddSub  mode=Addition  use_carryin=off  use_carryout=off  en=on  latency=3  precision=Full  arith_type=Unsigned  n_bits=16  bin_pt=14  quantization=Truncate  overflow=Wrap  use_behavioral_HDL=off  hw_selection=Fabric  pipelined=off  dbl_ovrd=off  block_type=addsub
  AddSub2 : xbsIndex_r4/AddSub  mode=Addition  use_carryin=off  use_carryout=off  en=on  latency=3  precision=Full  arith_type=Unsigned  n_bits=16  bin_pt=14  quantization=Truncate  overflow=Wrap  use_behavioral_HDL=off  hw_selection=Fabric  pipelined=off  dbl_ovrd=off  block_type=addsub
  Delay : xbsIndex_r4/Delay  rst=off  infoeditControl=Selection of Reset will increase slice count due to use of real FFs and instead of SRLs  en=off  latency=3  reg_retiming=off  dbl_ovrd=off  block_type=delay
      settings: infoedit=Hardware notes: A delay line is a chain, each link of which is an SRL16 or SRL32 followed by a flip-flop.
  Delay1 : xbsIndex_r4/Delay  rst=off  infoeditControl=Selection of Reset will increase slice count due to use of real FFs and instead of SRLs  en=off  latency=3  reg_retiming=off  dbl_ovrd=off  block_type=delay
      settings: infoedit=Hardware notes: A delay line is a chain, each link of which is an SRL16 or SRL32 followed by a flip-flop.
  Terminator : Terminator
  Terminator1 : Terminator
  Terminator2 : Terminator
  Braw : Outport
  EnOut : Outport  Port=2
  wires:
  AddSub/1 -> AddSub1/1, Add0/1
  AddSub1/1 -> Add2/1, Braw/1
  Delay/1 -> EnOut/1
  Enable/1 -> AddSub2/3, AddSub/3, Delay1/1
  Sum1/1 -> AddSub/2
  Sum0/1 -> AddSub/1
  Delay1/1 -> Delay/1, AddSub1/3
  Add0/1 -> Terminator/1
  Add2/1 -> Terminator1/1
  AddSub2/1 -> Add1/1, AddSub1/2
  Sum2/1 -> AddSub2/1
  Coef_Offset/1 -> AddSub2/2
  Add1/1 -> Terminator2/1

== system SysGenBCM_MR0/DspCoreMr/Proc/ChargeBlk1/FloatingConvAndMult0 ==
  Enable : Inport  SampleTime=5.385E-9
  ADCsum0 : Inport  Port=2
  ScoefA : Inport  Port=3  SampleTime=5.385E-9
  Convert0 : xbsIndex_r4/Convert  gui_display_data_type=Fixed-point  arith_type="Signed  (2's comp)"  n_bits=32  bin_pt=0  float_type=Single  exp_bits=8  fraction_bits=24  quantization=Truncate  overflow=Wrap  en=on  latency=1  pipeline=off  dbl_ovrd=off  block_type=convert
  Convert1 : xbsIndex_r4/Convert  gui_display_data_type=Floating-point  arith_type=Floating-point  n_bits=16  bin_pt=14  float_type=Single  exp_bits=8  fraction_bits=24  quantization=Truncate  overflow=Wrap  en=off  latency=1  pipeline=off  dbl_ovrd=off  block_type=convert
  Delay : xbsIndex_r4/Delay  rst=off  infoeditControl=Selection of Reset will increase slice count due to use of real FFs and instead of SRLs  en=off  latency=6  reg_retiming=off  dbl_ovrd=off  block_type=delay
      settings: infoedit=Hardware notes: A delay line is a chain, each link of which is an SRL16 or SRL32 followed by a flip-flop.
  Mult : xbsIndex_r4/Mult  precision=Full  arith_type="Signed  (2's comp)"  n_bits=16  bin_pt=14  quantization=Truncate  overflow=Wrap  en=off  latency=4  use_behavioral_HDL=off  opt=Speed  use_embedded=on  optimum_pipeline=off  pipeline=on  dbl_ovrd=off  use_rpm=on  placement_style=Triangular  block_type=mult
  MultResult : xbsIndex_r4/Gateway Out  inherit_from_input=on  hdl_port=on  rows=1  columns=1  UseAsDAC=off  DACChannel='1'  interface=AXI4-Lite  automatic_assignment=off  address_offset=hex2dec('118')  intf_name=''  intf_description=''  timing_constraint=None  locs_specified=off  LOCs={}  io_standard={}  block_type=gatewayout
  Terminator : Terminator
  ResOut : Outport
  EnOut : Outport  Port=2
  wires:
  Mult/1 -> MultResult/1, ResOut/1
  Convert0/1 -> Convert1/1
  Enable/1 -> Delay/1, Convert0/2
  ScoefA/1 -> Mult/2
  Convert1/1 -> Mult/1
  Delay/1 -> EnOut/1
  ADCsum0/1 -> Convert0/1
  MultResult/1 -> Terminator/1

== system SysGenBCM_MR0/DspCoreMr/Proc/ChargeBlk1/FloatingConvAndMult1 ==
  Enable : Inport  SampleTime=5.385E-9
  ADCsum0 : Inport  Port=2
  ScoefA : Inport  Port=3  SampleTime=5.385E-9
  Convert0 : xbsIndex_r4/Convert  gui_display_data_type=Fixed-point  arith_type="Signed  (2's comp)"  n_bits=32  bin_pt=0  float_type=Single  exp_bits=8  fraction_bits=24  quantization=Truncate  overflow=Wrap  en=on  latency=1  pipeline=off  dbl_ovrd=off  block_type=convert
  Convert1 : xbsIndex_r4/Convert  gui_display_data_type=Floating-point  arith_type=Floating-point  n_bits=16  bin_pt=14  float_type=Single  exp_bits=8  fraction_bits=24  quantization=Truncate  overflow=Wrap  en=off  latency=1  pipeline=off  dbl_ovrd=off  block_type=convert
  Delay : xbsIndex_r4/Delay  rst=off  infoeditControl=Selection of Reset will increase slice count due to use of real FFs and instead of SRLs  en=off  latency=6  reg_retiming=off  dbl_ovrd=off  block_type=delay
      settings: infoedit=Hardware notes: A delay line is a chain, each link of which is an SRL16 or SRL32 followed by a flip-flop.
  Mult : xbsIndex_r4/Mult  precision=Full  arith_type="Signed  (2's comp)"  n_bits=16  bin_pt=14  quantization=Truncate  overflow=Wrap  en=off  latency=4  use_behavioral_HDL=off  opt=Speed  use_embedded=on  optimum_pipeline=off  pipeline=on  dbl_ovrd=off  use_rpm=on  placement_style=Triangular  block_type=mult
  MultResult : xbsIndex_r4/Gateway Out  inherit_from_input=on  hdl_port=on  rows=1  columns=1  UseAsDAC=off  DACChannel='1'  interface=AXI4-Lite  automatic_assignment=off  address_offset=hex2dec('11C')  intf_name=''  intf_description=''  timing_constraint=None  locs_specified=off  LOCs={}  io_standard={}  block_type=gatewayout
  Terminator : Terminator
  ResOut : Outport
  EnOut : Outport  Port=2
  wires:
  Mult/1 -> MultResult/1, ResOut/1
  Convert0/1 -> Convert1/1
  Enable/1 -> Delay/1, Convert0/2
  ScoefA/1 -> Mult/2
  Convert1/1 -> Mult/1
  Delay/1 -> EnOut/1
  ADCsum0/1 -> Convert0/1
  MultResult/1 -> Terminator/1

== system SysGenBCM_MR0/DspCoreMr/Proc/ChargeBlk1/FloatingConvAndMult2 ==
  Enable : Inport  SampleTime=5.385E-9
  ADCsum0 : Inport  Port=2
  ScoefA : Inport  Port=3  SampleTime=5.385E-9
  Convert0 : xbsIndex_r4/Convert  gui_display_data_type=Fixed-point  arith_type="Signed  (2's comp)"  n_bits=32  bin_pt=0  float_type=Single  exp_bits=8  fraction_bits=24  quantization=Truncate  overflow=Wrap  en=on  latency=1  pipeline=off  dbl_ovrd=off  block_type=convert
  Convert1 : xbsIndex_r4/Convert  gui_display_data_type=Floating-point  arith_type=Floating-point  n_bits=16  bin_pt=14  float_type=Single  exp_bits=8  fraction_bits=24  quantization=Truncate  overflow=Wrap  en=off  latency=1  pipeline=off  dbl_ovrd=off  block_type=convert
  Delay : xbsIndex_r4/Delay  rst=off  infoeditControl=Selection of Reset will increase slice count due to use of real FFs and instead of SRLs  en=off  latency=6  reg_retiming=off  dbl_ovrd=off  block_type=delay
      settings: infoedit=Hardware notes: A delay line is a chain, each link of which is an SRL16 or SRL32 followed by a flip-flop.
  Mult : xbsIndex_r4/Mult  precision=Full  arith_type="Signed  (2's comp)"  n_bits=16  bin_pt=14  quantization=Truncate  overflow=Wrap  en=off  latency=4  use_behavioral_HDL=off  opt=Speed  use_embedded=on  optimum_pipeline=off  pipeline=on  dbl_ovrd=off  use_rpm=on  placement_style=Triangular  block_type=mult
  MultResult : xbsIndex_r4/Gateway Out  inherit_from_input=on  hdl_port=on  rows=1  columns=1  UseAsDAC=off  DACChannel='1'  interface=AXI4-Lite  automatic_assignment=off  address_offset=hex2dec('120')  intf_name=''  intf_description=''  timing_constraint=None  locs_specified=off  LOCs={}  io_standard={}  block_type=gatewayout
  Terminator : Terminator
  ResOut : Outport
  EnOut : Outport  Port=2
  wires:
  Mult/1 -> MultResult/1, ResOut/1
  Convert0/1 -> Convert1/1
  Enable/1 -> Delay/1, Convert0/2
  ScoefA/1 -> Mult/2
  Convert1/1 -> Mult/1
  Delay/1 -> EnOut/1
  ADCsum0/1 -> Convert0/1
  MultResult/1 -> Terminator/1

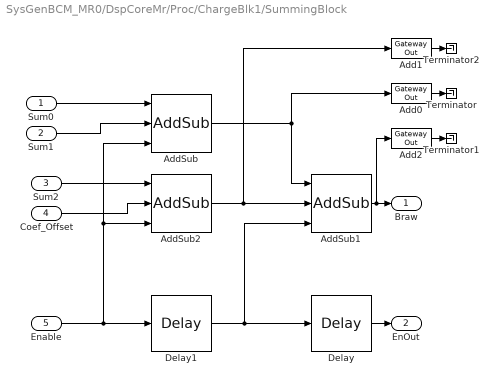
== system SysGenBCM_MR0/DspCoreMr/Proc/ChargeBlk1/SummingBlock ==
  Sum0 : Inport
  Sum1 : Inport  Port=2
  Sum2 : Inport  Port=3
  Coef_Offset : Inport  Port=4
  Enable : Inport  Port=5
  Add0 : xbsIndex_r4/Gateway Out  inherit_from_input=on  hdl_port=on  rows=1  columns=1  UseAsDAC=off  DACChannel='1'  interface=AXI4-Lite  automatic_assignment=off  address_offset=hex2dec('124')  intf_name=''  intf_description=''  timing_constraint=None  locs_specified=off  LOCs={}  io_standard={}  block_type=gatewayout
  Add1 : xbsIndex_r4/Gateway Out  inherit_from_input=on  hdl_port=on  rows=1  columns=1  UseAsDAC=off  DACChannel='1'  interface=AXI4-Lite  automatic_assignment=off  address_offset=hex2dec('128')  intf_name=''  intf_description=''  timing_constraint=None  locs_specified=off  LOCs={}  io_standard={}  block_type=gatewayout
  Add2 : xbsIndex_r4/Gateway Out  inherit_from_input=on  hdl_port=on  rows=1  columns=1  UseAsDAC=off  DACChannel='1'  interface=AXI4-Lite  automatic_assignment=off  address_offset=hex2dec('12c')  intf_name=''  intf_description=''  timing_constraint=None  locs_specified=off  LOCs={}  io_standard={}  block_type=gatewayout
  AddSub : xbsIndex_r4/AddSub  mode=Addition  use_carryin=off  use_carryout=off  en=on  latency=3  precision=Full  arith_type=Unsigned  n_bits=16  bin_pt=14  quantization=Truncate  overflow=Wrap  use_behavioral_HDL=off  hw_selection=Fabric  pipelined=off  dbl_ovrd=off  block_type=addsub
  AddSub1 : xbsIndex_r4/AddSub  mode=Addition  use_carryin=off  use_carryout=off  en=on  latency=3  precision=Full  arith_type=Unsigned  n_bits=16  bin_pt=14  quantization=Truncate  overflow=Wrap  use_behavioral_HDL=off  hw_selection=Fabric  pipelined=off  dbl_ovrd=off  block_type=addsub
  AddSub2 : xbsIndex_r4/AddSub  mode=Addition  use_carryin=off  use_carryout=off  en=on  latency=3  precision=Full  arith_type=Unsigned  n_bits=16  bin_pt=14  quantization=Truncate  overflow=Wrap  use_behavioral_HDL=off  hw_selection=Fabric  pipelined=off  dbl_ovrd=off  block_type=addsub
  Delay : xbsIndex_r4/Delay  rst=off  infoeditControl=Selection of Reset will increase slice count due to use of real FFs and instead of SRLs  en=off  latency=3  reg_retiming=off  dbl_ovrd=off  block_type=delay
      settings: infoedit=Hardware notes: A delay line is a chain, each link of which is an SRL16 or SRL32 followed by a flip-flop.
  Delay1 : xbsIndex_r4/Delay  rst=off  infoeditControl=Selection of Reset will increase slice count due to use of real FFs and instead of SRLs  en=off  latency=3  reg_retiming=off  dbl_ovrd=off  block_type=delay
      settings: infoedit=Hardware notes: A delay line is a chain, each link of which is an SRL16 or SRL32 followed by a flip-flop.
  Terminator : Terminator
  Terminator1 : Terminator
  Terminator2 : Terminator
  Braw : Outport
  EnOut : Outport  Port=2
  wires:
  AddSub/1 -> AddSub1/1, Add0/1
  AddSub1/1 -> Add2/1, Braw/1
  Delay/1 -> EnOut/1
  Enable/1 -> AddSub2/3, AddSub/3, Delay1/1
  Sum1/1 -> AddSub/2
  Sum0/1 -> AddSub/1
  Delay1/1 -> Delay/1, AddSub1/3
  Add0/1 -> Terminator/1
  Add2/1 -> Terminator1/1
  AddSub2/1 -> Add1/1, AddSub1/2
  Sum2/1 -> AddSub2/1
  Coef_Offset/1 -> AddSub2/2
  Add1/1 -> Terminator2/1
